simulink model "CE_AMP_TB_YT"  (R2022a)
settings: Solver=VariableStepAuto  StartTime=0.0  StopTime=.25  RelTol=1e-4
libraries: fl_lib x6, nesl_utility x4, dsparch4 x1, ce_amp_ckt_lib x1
settings Model: SimulationMode=accelerator  Creator=kschutz  LastModifiedBy=kschutz
settings SolverCC: AlgebraicLoopSolver=TrustRegion
settings DebuggingCC: UnconnectedInputMsg=warning  UnconnectedOutputMsg=warning  UnconnectedLineMsg=warning  SFMachineParentedDataDiag=warning
settings RTWCC: DLArmComputeVersion=19.05

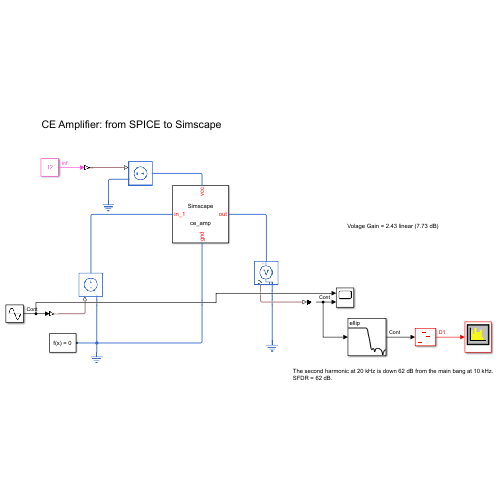
[thumbnail: Simulink's stored preview of the top-level diagram]
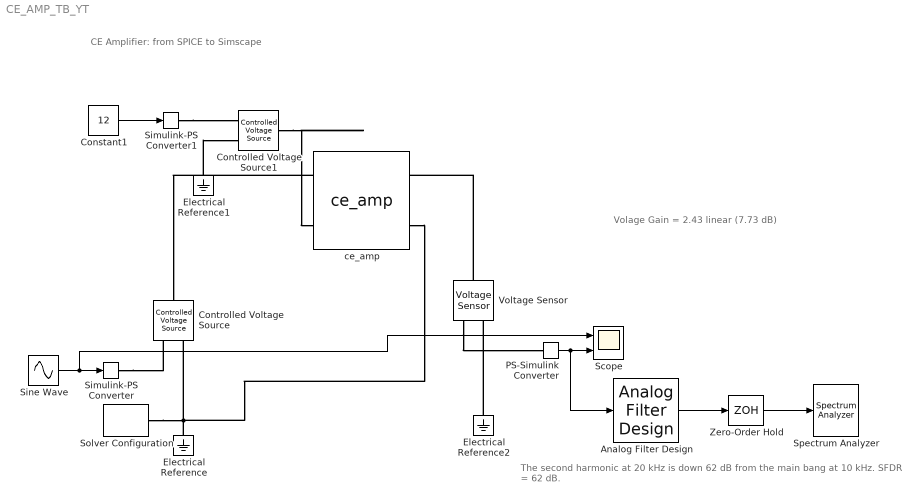
== system CE_AMP_TB_YT ==
  note: The second harmonic at 20 kHz is down 62 dB from the main bang at 10 kHz.
      | SFDR = 62 dB.
  note: Volage Gain = 2.43 linear (7.73 dB)
  note: CE Amplifier: from SPICE to Simscape
  Analog Filter Design : dsparch4/Analog Filter Design  method=Elliptic  filttype=Lowpass  N=8  Wlo=2*pi*50e3  Whi=80  Rp=1  Rs=100
  Constant1 : Constant  Value=12
  Controlled Voltage Source : fl_lib/Electrical/Electrical Sources/Controlled Voltage Source
      settings: SourceProductBaseCode=PW,SS,VE
  Controlled Voltage Source1 : fl_lib/Electrical/Electrical Sources/Controlled Voltage Source
      settings: SourceProductBaseCode=PW,SS,VE
  Electrical Reference : fl_lib/Electrical/Electrical Elements/Electrical Reference
      settings: SourceProductBaseCode=PW,SS,VE
  Electrical Reference1 : fl_lib/Electrical/Electrical Elements/Electrical Reference
      settings: SourceProductBaseCode=PW,SS,VE
  Electrical Reference2 : fl_lib/Electrical/Electrical Elements/Electrical Reference
      settings: SourceProductBaseCode=PW,SS,VE
  PS-Simulink Converter : nesl_utility/PS-Simulink Converter  PhysicalDomain=network_engine_domain  SubClassName=ps_output  LeftPortType=input  RightPortType=output  PseudoPeriodic=off  Frequencies=[]  VectorFormat=1-D array  Unit=inherit  AffineConversion=off
      settings: SourceProductBaseCode=SS,PW,VE
  Scope : Scope  NumInputPorts=2
  Simulink-PS Converter : nesl_utility/Simulink-PS Converter  PhysicalDomain=network_engine_domain  SubClassName=ps_input  LeftPortType=input  RightPortType=output  PseudoPeriodic=off  Frequencies=[]  NoiseDistribution=none  NoiseParameters=[]  Unit=1  AffineConversion=off  FilteringAndDerivatives=provide  SimscapeFilterOrder=1  InputFilterTimeConstant=0.001  UdotUserProvided=0
      settings: SourceProductBaseCode=SS,PW,VE
  Simulink-PS Converter1 : nesl_utility/Simulink-PS Converter  PhysicalDomain=network_engine_domain  SubClassName=ps_input  LeftPortType=input  RightPortType=output  PseudoPeriodic=off  Frequencies=[]  NoiseDistribution=none  NoiseParameters=[]  Unit=1  AffineConversion=off  FilteringAndDerivatives=provide  SimscapeFilterOrder=1  InputFilterTimeConstant=0.001  UdotUserProvided=0
      settings: SourceProductBaseCode=SS,PW,VE
  Sine Wave : Sin  Amplitude=.2  Frequency=2*pi*10e3  SampleTime=0
  Solver Configuration : nesl_utility/Solver Configuration  PhysicalDomain=network_engine_domain  SubClassName=solver  LeftPortType=input  RightPortType=generic  Tones=[]  Harmonics=[]  SimulateNoise=off  Profile=off  UseLocalSampling=off  EnableSwitchedLinearOptims=on  FrequencyDomain=off  UseCCode=off  RelTol=0.001  AbsTol=1e-06  MinStep=1e-09  ToWorkspace=off  RevertToSquareIcSolve=off  NumHomotopyIterations=100  PhasorMode=off  PhasorModeNumHarmonics=1  IndexReductionMethod=DerivativeReplacement  DoDC=off  ResidualTolerance=1e-09  UseLocalSolver=off  LocalSolverChoice=NE_BACKWARD_EULER_ADVANCER  LocalSolverSampleTime=0.001  DoFixedCost=off  MaxNonlinIter=3  MaxModeIter=2  ComputeImpulses=off  ImpulseIterations=2  LinearAlgebra=auto  LinearAlgebraNumThread=0  EquationFormulation=NE_TIME_EF  DelaysMemoryBudget=1024  AutomaticFiltering=on  FilteringTimeConstant=0.001  PartitionStorageMethod=AS_NEEDED  PartitionMemoryBudget=1024  PartitionMethod=ROBUST
      settings: SourceProductBaseCode=SS,PW,VE
  Spectrum Analyzer : SpectrumAnalyzer
  Voltage Sensor : fl_lib/Electrical/Electrical Sensors/Voltage Sensor
      settings: SourceProductBaseCode=PW,SS,VE
  Zero-Order Hold : ZeroOrderHold  SampleTime=1/150e3
  ce_amp : ce_amp_ckt_lib/ce_amp  specifyParasiticValues=ee.enum.include.no  capacitorSeriesResistance=0 Ohm
      settings: InternalSimscapePortConfiguration="{\"Bottom\":[{\"id\":\"gnd\",\"label\":\"gnd\",\"type\":\"foundation.electrical.electrical\"}],\"Left\":[{\"id\":\"in_1\",\"label\":\"in_1\",\"type\":\"foundation.electrical.electrical\"}],\"Right\":[{\"id\":\"out\",\"label\":\"out\",\"type\":\"foundation.electrical.electrical\"}],\"Top\":[{\"id\":\"vcc\",\"label\":\"vcc\",\"type\":\"foundation.electrical.electrical\"}]}"
  wires:
  Constant1/1 -> Simulink-PS Converter1/1
  PS-Simulink Converter/1 -> Analog Filter Design/1, Scope/2
  Sine Wave/1 -> Scope/1, Simulink-PS Converter/1
  Zero-Order Hold/1 -> Spectrum Analyzer/1
  Analog Filter Design/1 -> Zero-Order Hold/1
  connections:
  Electrical Reference/LConn1 -- Solver Configuration/RConn1 -- ce_amp/RConn2 -- Controlled Voltage Source/RConn2
  Simulink-PS Converter/RConn1 -- Controlled Voltage Source/RConn1
  Electrical Reference1/LConn1 -- Controlled Voltage Source1/RConn2
  Simulink-PS Converter1/RConn1 -- Controlled Voltage Source1/RConn1
  Electrical Reference2/LConn1 -- Voltage Sensor/RConn2
  Voltage Sensor/RConn1 -- PS-Simulink Converter/LConn1
  ce_amp/LConn1 -- Controlled Voltage Source/LConn1
  Controlled Voltage Source1/LConn1 -- ce_amp/LConn2
  Voltage Sensor/LConn1 -- ce_amp/RConn1
